simulink model "model1"  (R2022b)
settings: Solver=VariableStepAuto  StartTime=0.0  StopTime=5  RelTol=1e-3
model workspace (MAT data in the model file):
  CC = [-1 -1]
undefined symbols (not defined in the file or in its folder): sigbuilder_block
libraries: simulink x1
settings Model: Creator=Administrator  LastModifiedBy=NINGMEI

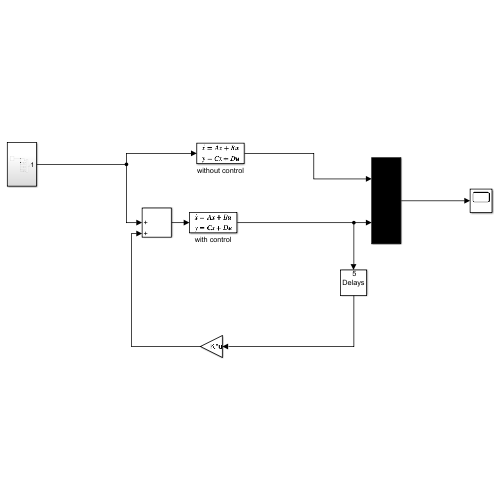
[thumbnail: Simulink's stored preview of the top-level diagram]
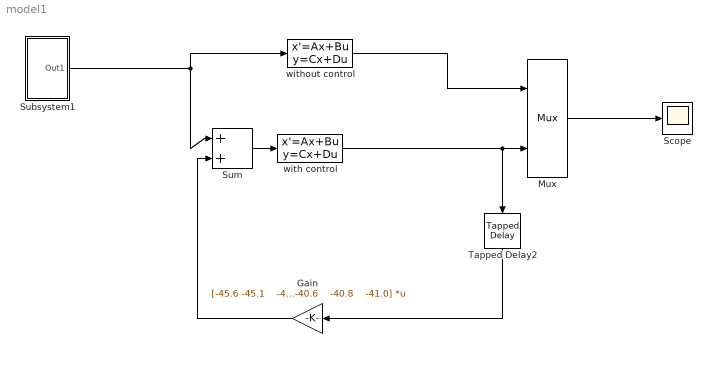
== system model1 ==
  Gain : Gain  Gain=|  Multiplication=Matrix(K*u)
      | [-45.6 -45.1    -44.7    -44.2    -43.7    -43.3
      | -52.3  -52.1    -51.9    -51.7    -51.5    -51.3 
      | -34.0  -33.7    -33.3    -33.0    -32.6    -32.3
      | -41.4    -41.2    -41.0    -40.8    -40.6    -40.4
      | -48.3    -48.2    -48.1    -48.1    -48.0    -47.9
      | -40.2    -40.3    -40.5    -40.6    -40.8    -41.0]
  Mux : Mux  Inputs=2
  Scope : Scope
  Subsystem1 : Subsystem
  Sum : Sum  Inputs=|++
  Tapped Delay2 : simulink/Discrete/Tapped Delay  vinit=0.0  samptime=0.001  NumDelays=5  DelayOrder=Oldest  includeCurrent=on
  with control : StateSpace  A=|  B=eye(6)  C=[1,0,0,0,0,0]  D=zeros(1,6)  InitialCondition=0
      | [-5 2 3 0 0 0
      | 2 -6 0 0 1 3
      | 3 0 -5 2 0 0
      | 0 0 2 -2 0 0
      | 0 1 0 0 -4 3
      | 0 3 0 0 3 -6]
  without control : StateSpace  A=|  B=eye(6)  C=[1,0,0,0,0,0]  D=zeros(1,6)  InitialCondition=0
      | [-5 2 3 0 0 0
      | 2 -6 0 0 1 3
      | 3 0 -5 2 0 0
      | 0 0 2 -2 0 0
      | 0 1 0 0 -4 3
      | 0 3 0 0 3 -6]
  wires:
  without control/1 -> Mux/1
  Gain/1 -> Sum/2
  Mux/1 -> Scope/1
  with control/1 -> Mux/2, Tapped Delay2/1
  Tapped Delay2/1 -> Gain/1
  Subsystem1/1(Out1) -> without control/1, Sum/1
  Sum/1 -> with control/1

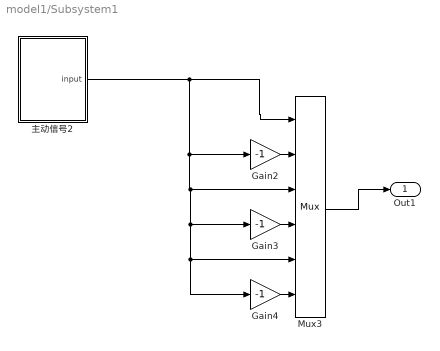
== system model1/Subsystem1 ==
  Gain2 : Gain  Gain=-1
  Gain3 : Gain  Gain=-1
  Gain4 : Gain  Gain=-1
  Mux3 : Mux  Inputs=6
  主动信号2 : Subsystem
  Out1 : Outport
  wires:
  Mux3/1 -> Out1/1
  Gain2/1 -> Mux3/2
  Gain3/1 -> Mux3/4
  Gain4/1 -> Mux3/6
  主动信号2/1(input) -> Gain4/1, Mux3/5, Gain3/1, Mux3/3, Gain2/1, Mux3/1

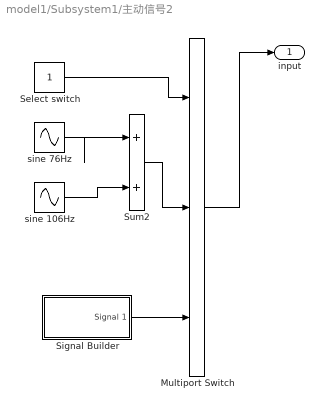
== system model1/Subsystem1/主动信号2 ==
  Multiport Switch : MultiPortSwitch  Inputs=2  SaturateOnIntegerOverflow=off  InputSameDT=off
  Select switch : Constant
  Signal Builder : Subsystem  Tag=STV Subsys  LoadFcn=sigbuilder_block('load');  StartFcn=sigbuilder_block('start');  StopFcn=sigbuilder_block('stop');  ClipboardFcn=sigbuilder_block('clipboard');  mask(Sigbuilder block){tuvar=[0:10]}
      mask help: Simulink:masks:SigbuilderBlock_MD
      mask init:
      | if ~strcmp(get_param(bdroot(gcbh),'SimulationStatus'),'stopped') tuvar = sigbuilder_block('maskInit'); end
      settings: CopyFcn=sigbuilder_block('copy');  DeleteFcn=sigbuilder_block('delete');  ModelCloseFcn=sigbuilder_block('modelClose');  PreSaveFcn=sigbuilder_block('preSave');  PauseFcn=sigbuilder_block('pause');  ContinueFcn=sigbuilder_block('continue');  NameChangeFcn=sigbuilder_block('namechange');  OpenFcn=sigbuilder_block('open',[230.897 85.6552 549.931 396.621 ]);  CloseFcn=sigbuilder_block('close');
      mask Display: plot(0, 0, 100, 100,[2, 2, 32, 32, 2], [68, 8, 8, 68, 68],[32, 2], [38, 38], [32, 19, 2],[53, 60, 44], [32, 17, 17, 2],[16, 16, 31, 31]);txt = getActiveGroup(gcbh);text(2, 100, txt,'verticalAlignment', 'top');
  Sum2 : Sum  Inputs=|++
  sine 106Hz : Sin  Amplitude=5  Frequency=2*pi*1.06  SampleTime=0
  sine 76Hz : Sin  Amplitude=5  Frequency=2*pi*0.76  SampleTime=0
  input : Outport
  wires:
  Select switch/1 -> Multiport Switch/1
  sine 76Hz/1 -> Sum2/1
  Multiport Switch/1 -> input/1
  Signal Builder/1(Signal 1) -> Multiport Switch/3
  sine 106Hz/1 -> Sum2/2
  Sum2/1 -> Multiport Switch/2

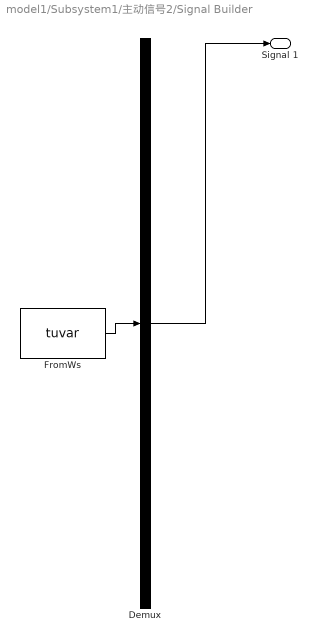
== system model1/Subsystem1/主动信号2/Signal Builder ==
  Demux : Demux  Tag=STV Demux  Outputs=1
      settings: DisplayOption=none
  FromWs : FromWorkspace  Tag=STV FromWs  VariableName=tuvar
      SigBuilderData=|
      | common.afterFinalStr = 'Extrapolate'
      | common.sampleTime = 0
      | dataSet.timeRange = [0 10]
      | dataSet.name = 'Group 1'
      | sbobj.Groups.Name = 'Group 1'
      | sbobj.Groups.Signals.Name = 'Signal 1'
      | sbobj.Groups.Signals.XData = [0 0.1 0.1 0.1001 0.1001 10]
      | sbobj.Groups.Signals.YData = [0 0 1 1 0 0]
  Signal 1 : Outport  Tag=STV Outport
  wires:
  Demux/1 -> Signal 1/1
  FromWs/1 -> Demux/1
